simulink model "Wind_turbine_model_L"  (R2020a)
settings: Solver=daessc  StartTime=0.0  StopTime=70  RelTol=1e-3
model workspace (MAT data in the model file):
  Tw : Simulink.Parameter (value not decoded)
  c : Simulink.Parameter (value not decoded)
  r : Simulink.Parameter (value not decoded)
values from neighbouring files (symbols this model uses):
  a1 = 0.5176    [data.mat]
  a2 = 116    [data.mat]
  a3 = 0.4    [data.mat]
  a4 = 5    [data.mat]
  a5 = 21    [data.mat]
  a6 = 0.0068    [data.mat]
  a7 = 0.09    [data.mat]
  a8 = 0.035    [data.mat]
  Ad = 6031.85789489    [data.mat]
  D = 1e-3    (= 0.001)    [Generator_specs.m]
  denp = den_P    [Wind_Turbine_Pitch.m]    (also in data.mat = [91260000000000 145900000000000 1.431e+17 7.554e+15 2.279e+1)
  dent = den_P    [Wind_Turbine_Pitch.m]    (also in data.mat = [91260000000000 145900000000000 1.431e+17 7.554e+15 2.279e+1)
  f = 50    [Generator_specs.m]
  Fs = Vs*sqrt(2/3)/(2*pi*f)    [Generator_specs.m]
  fsw = 4e3    (= 4000)    [Generator_specs.m]
  J = 127/2    (= 63.5)    [Generator_specs.m]
  ki_id = (wn1^2)*Lr*sigma    (= 491.599501999)    [Generator_specs.m]
  ki_n = ((wnn^2)*J)/p    (= 203200)    [Generator_specs.m]
  Kopt = ((0.5*ro*pi*(Radius^5)*cp_max)/(lambda_opt^3))    (= 227539.221001)    [Generator_specs.m]
  kp_id = (2*wn1*sigma*Lr)-Rr    (= 0.5771)    [Generator_specs.m]
  kp_n = (2*wnn*J)/p    (= 5080)    [Generator_specs.m]
  Lm = 2.5e-3    (= 0.0025)    [Generator_specs.m]
  Lr = Lm + Lsi    (= 0.002587)    [Generator_specs.m]
  Ls = Lm + Lsi    (= 0.002587)    [Generator_specs.m]
  Lsi = 0.087e-3    (= 8.7e-05)    [Generator_specs.m]
  N = 100    [Generator_specs.m]
  nump = num_P    [Wind_Turbine_Pitch.m]    (also in data.mat = [16590000 26450000 25540000000 6335000000 3680000000000])
  numt = num_T    [Wind_Turbine_Pitch.m]    (also in data.mat = [-75000000 -527900000000 -306700000000000])
  p = 2    [Generator_specs.m]
  Ps = 2e6    (= 2000000)    [Generator_specs.m]
  Rr = 2.9e-3    (= 0.0029)    [Generator_specs.m]
  Rs = 2.6e-3    (= 0.0026)    [Generator_specs.m]
  s = tf('s')    [Wind_Turbine_Pitch.m]
  sigma = 1 - Lm^2/(Ls*Lr)    (= 0.0661284179513)    [Generator_specs.m]    (also in data.mat = 0.075)
  Tem = 12732    [Generator_specs.m]
  Tgd_max = 14000    [Wind_Turbine_Pitch.m]    (also in data.mat)
  Tie = 1    [data.mat]
  Tiu = 10000    [data.mat]
  Tix = 1    [data.mat]
  Tpe = 1    [data.mat]
  Tpu = 10000    [data.mat]
  Tpx = 10000    [data.mat]
  Ts = 1/fsw/50    (= 5e-06)    [Generator_specs.m]
  Vbus = Vr_stator*sqrt(2)    [Generator_specs.m]
  Vs = 690    [Generator_specs.m]
  WT_Params =     [data.mat]
symbols that are objects in the model workspace (value not decoded): c, r, Tw
undefined symbols (not defined in the file or in its folder): DiscIntNeverNeededParam, sigbuilder_block, X, Y, Z
libraries: sm_lib x21, fl_lib x18, nesl_utility x18, powerlib x8, sdl_lib x3, powerlib_meascontrol x1
(part 2 of 3)

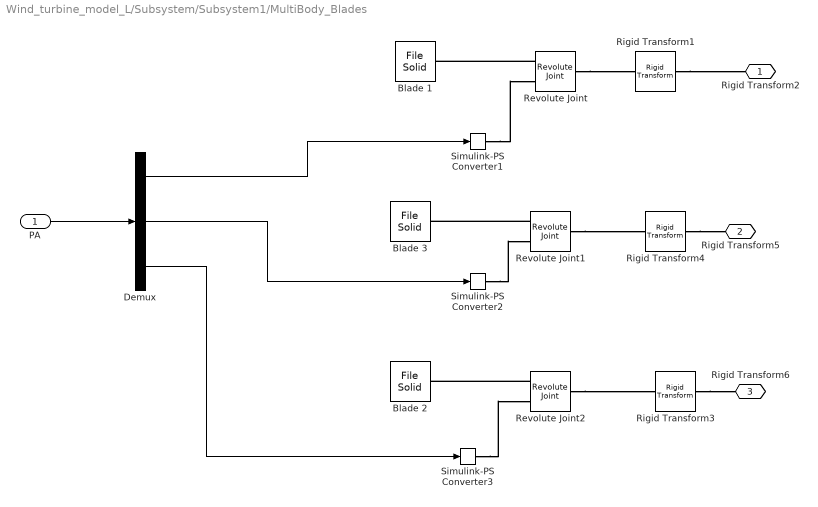
== system Wind_turbine_model_L/Subsystem/Subsystem1/MultiBody_Blades ==
  PA : Inport
  Blade 1 : sm_lib/Body Elements/File Solid  ExtGeomFileName=F:\Altran_Documents\Pilot_Project\Wind_energy\Wind_Turbine_MBSE\Local_WIP\WT blade.STEP  UnitType=FromFile  ExtGeomFileUnits=m  StepReaderType=HEX  ExportConvexHullGeometry=off  InertiaType=PointMass  Mass=5388  MassUnits=kg  CenterOfMass=[0 0 0]  CenterOfMassUnits=m  MomentsOfInertia=[1 1 1]  MomentsOfInertiaUnits=kg*m^2  ProductsOfInertia=[0 0 0]  ProductsOfInertiaUnits=kg*m^2  BasedOnType=DensityFromFile  Density=1000  DensityUnits=kg/m^3  DoExposeReferenceFrame=on  SerializedFrames=<Frames/>  GraphicType=FromGeometry  MarkerShape=Sphere  MarkerSize=10  GraphicVisPropType=SimpleVisualProperties  GraphicDiffuseColor=[0.5 0.5 0.5]  GraphicSpecularColor=[0.5 0.5 0.5 1.0]  GraphicAmbientColor=[0.15 0.15 0.15 1.0]  GraphicEmissiveColor=[0.0 0.0 0.0 1.0]  GraphicShininess=75  GraphicOpacity=1.0
  Blade 2 : sm_lib/Body Elements/File Solid  ExtGeomFileName=F:\Altran_Documents\Pilot_Project\Wind_energy\Wind_Turbine_MBSE\Local_WIP\WT blade.STEP  UnitType=FromFile  ExtGeomFileUnits=m  StepReaderType=HEX  ExportConvexHullGeometry=off  InertiaType=PointMass  Mass=5388  MassUnits=kg  CenterOfMass=[0 0 0]  CenterOfMassUnits=m  MomentsOfInertia=[1 1 1]  MomentsOfInertiaUnits=kg*m^2  ProductsOfInertia=[0 0 0]  ProductsOfInertiaUnits=kg*m^2  BasedOnType=DensityFromFile  Density=1000  DensityUnits=kg/m^3  DoExposeReferenceFrame=on  SerializedFrames=<Frames/>  GraphicType=FromGeometry  MarkerShape=Sphere  MarkerSize=10  GraphicVisPropType=SimpleVisualProperties  GraphicDiffuseColor=[0.5 0.5 0.5]  GraphicSpecularColor=[0.5 0.5 0.5 1.0]  GraphicAmbientColor=[0.15 0.15 0.15 1.0]  GraphicEmissiveColor=[0.0 0.0 0.0 1.0]  GraphicShininess=75  GraphicOpacity=1.0
  Blade 3 : sm_lib/Body Elements/File Solid  ExtGeomFileName=F:\Altran_Documents\Pilot_Project\Wind_energy\Wind_Turbine_MBSE\Local_WIP\WT blade.STEP  UnitType=FromFile  ExtGeomFileUnits=m  StepReaderType=HEX  ExportConvexHullGeometry=off  InertiaType=PointMass  Mass=5388  MassUnits=kg  CenterOfMass=[0 0 0]  CenterOfMassUnits=m  MomentsOfInertia=[1 1 1]  MomentsOfInertiaUnits=kg*m^2  ProductsOfInertia=[0 0 0]  ProductsOfInertiaUnits=kg*m^2  BasedOnType=DensityFromFile  Density=1000  DensityUnits=kg/m^3  DoExposeReferenceFrame=on  SerializedFrames=<Frames/>  GraphicType=FromGeometry  MarkerShape=Sphere  MarkerSize=10  GraphicVisPropType=SimpleVisualProperties  GraphicDiffuseColor=[0.5 0.5 0.5]  GraphicSpecularColor=[0.5 0.5 0.5 1.0]  GraphicAmbientColor=[0.15 0.15 0.15 1.0]  GraphicEmissiveColor=[0.0 0.0 0.0 1.0]  GraphicShininess=75  GraphicOpacity=1.0
  Demux : Demux  Outputs=3
  Revolute Joint : sm_lib/Joints/Revolute Joint  JointMode=Normal  SenseConstraintForce=off  SenseConstraintForceX=off  SenseConstraintForceY=off  SenseConstraintForceZ=off  SenseConstraintTorque=off  SenseConstraintTorqueX=off  SenseConstraintTorqueY=off  SenseConstraintTorqueZ=off  SenseTotalForce=off  SenseTotalForceX=off  SenseTotalForceY=off  SenseTotalForceZ=off  SenseTotalTorque=off  SenseTotalTorqueX=off  SenseTotalTorqueY=off  SenseTotalTorqueZ=off  CompositeWrenchDir=BaseOnFollower  CompositeWrenchFrame=BaseFrame  EquilibriumPosition=0  EquilibriumPositionUnits=deg  SpringStiffness=0  SpringStiffnessUnits=N*m/deg  DampingCoefficient=0  DampingCoefficientUnits=N*m/(deg/s)  TorqueActuationMode=ComputedTorque  MotionActuationMode=InputMotion  SensePosition=off  SenseVelocity=off  SenseAcceleration=off  SenseTorqueForce=off  SenseLowerLimitTorqueForce=off  SenseUpperLimitTorqueForce=off  LowerLimitSpecify=off  LowerLimitBound=-90  LowerLimitBoundUnits=deg  LowerLimitStiffness=1e4  LowerLimitStiffnessUnits=N*m/deg  LowerLimitDamping=10  LowerLimitDampingUnits=N*m/(deg/s)  LowerLimitTransitionRegionWidth=0.1  LowerLimitTransitionRegionWidthUnits=deg  UpperLimitSpecify=off  UpperLimitBound=90  UpperLimitBoundUnits=deg  UpperLimitStiffness=1e4  UpperLimitStiffnessUnits=N*m/deg  UpperLimitDamping=10  UpperLimitDampingUnits=N*m/(deg/s)  UpperLimitTransitionRegionWidth=0.1  UpperLimitTransitionRegionWidthUnits=deg  PositionTargetSpecify=off  PositionTargetPriority=High  PositionTargetValue=30  PositionTargetValueUnits=deg  VelocityTargetSpecify=off  VelocityTargetPriority=High  VelocityTargetValue=0  VelocityTargetValueUnits=deg/s
  Revolute Joint1 : sm_lib/Joints/Revolute Joint  JointMode=Normal  SenseConstraintForce=off  SenseConstraintForceX=off  SenseConstraintForceY=off  SenseConstraintForceZ=off  SenseConstraintTorque=off  SenseConstraintTorqueX=off  SenseConstraintTorqueY=off  SenseConstraintTorqueZ=off  SenseTotalForce=off  SenseTotalForceX=off  SenseTotalForceY=off  SenseTotalForceZ=off  SenseTotalTorque=off  SenseTotalTorqueX=off  SenseTotalTorqueY=off  SenseTotalTorqueZ=off  CompositeWrenchDir=BaseOnFollower  CompositeWrenchFrame=BaseFrame  EquilibriumPosition=0  EquilibriumPositionUnits=deg  SpringStiffness=0  SpringStiffnessUnits=N*m/deg  DampingCoefficient=0  DampingCoefficientUnits=N*m/(deg/s)  TorqueActuationMode=ComputedTorque  MotionActuationMode=InputMotion  SensePosition=off  SenseVelocity=off  SenseAcceleration=off  SenseTorqueForce=off  SenseLowerLimitTorqueForce=off  SenseUpperLimitTorqueForce=off  LowerLimitSpecify=off  LowerLimitBound=-90  LowerLimitBoundUnits=deg  LowerLimitStiffness=1e4  LowerLimitStiffnessUnits=N*m/deg  LowerLimitDamping=10  LowerLimitDampingUnits=N*m/(deg/s)  LowerLimitTransitionRegionWidth=0.1  LowerLimitTransitionRegionWidthUnits=deg  UpperLimitSpecify=off  UpperLimitBound=90  UpperLimitBoundUnits=deg  UpperLimitStiffness=1e4  UpperLimitStiffnessUnits=N*m/deg  UpperLimitDamping=10  UpperLimitDampingUnits=N*m/(deg/s)  UpperLimitTransitionRegionWidth=0.1  UpperLimitTransitionRegionWidthUnits=deg  PositionTargetSpecify=off  PositionTargetPriority=High  PositionTargetValue=30  PositionTargetValueUnits=deg  VelocityTargetSpecify=off  VelocityTargetPriority=High  VelocityTargetValue=0  VelocityTargetValueUnits=deg/s
  Revolute Joint2 : sm_lib/Joints/Revolute Joint  JointMode=Normal  SenseConstraintForce=off  SenseConstraintForceX=off  SenseConstraintForceY=off  SenseConstraintForceZ=off  SenseConstraintTorque=off  SenseConstraintTorqueX=off  SenseConstraintTorqueY=off  SenseConstraintTorqueZ=off  SenseTotalForce=off  SenseTotalForceX=off  SenseTotalForceY=off  SenseTotalForceZ=off  SenseTotalTorque=off  SenseTotalTorqueX=off  SenseTotalTorqueY=off  SenseTotalTorqueZ=off  CompositeWrenchDir=BaseOnFollower  CompositeWrenchFrame=BaseFrame  EquilibriumPosition=0  EquilibriumPositionUnits=deg  SpringStiffness=0  SpringStiffnessUnits=N*m/deg  DampingCoefficient=0  DampingCoefficientUnits=N*m/(deg/s)  TorqueActuationMode=ComputedTorque  MotionActuationMode=InputMotion  SensePosition=off  SenseVelocity=off  SenseAcceleration=off  SenseTorqueForce=off  SenseLowerLimitTorqueForce=off  SenseUpperLimitTorqueForce=off  LowerLimitSpecify=off  LowerLimitBound=-90  LowerLimitBoundUnits=deg  LowerLimitStiffness=1e4  LowerLimitStiffnessUnits=N*m/deg  LowerLimitDamping=10  LowerLimitDampingUnits=N*m/(deg/s)  LowerLimitTransitionRegionWidth=0.1  LowerLimitTransitionRegionWidthUnits=deg  UpperLimitSpecify=off  UpperLimitBound=90  UpperLimitBoundUnits=deg  UpperLimitStiffness=1e4  UpperLimitStiffnessUnits=N*m/deg  UpperLimitDamping=10  UpperLimitDampingUnits=N*m/(deg/s)  UpperLimitTransitionRegionWidth=0.1  UpperLimitTransitionRegionWidthUnits=deg  PositionTargetSpecify=off  PositionTargetPriority=High  PositionTargetValue=30  PositionTargetValueUnits=deg  VelocityTargetSpecify=off  VelocityTargetPriority=High  VelocityTargetValue=0  VelocityTargetValueUnits=deg/s
  Rigid Transform1 : sm_lib/Frames and Transforms/Rigid Transform  TranslationMethod=StandardAxis  TranslationStandardOffset=3.5  TranslationLengthUnit=m  TranslationStandardAxis=+Z  TranslationCartesianOffset=[0 0 0]  TranslationROffset=0  TranslationROffsetUnits=m  TranslationZOffset=0  TranslationZOffsetUnits=m  TranslationThetaOffset=0  TranslationThetaOffsetUnits=deg  RotationMethod=StandardAxis  RotationAngleUnits=deg  RotationStandardAxis=+Z  RotationAngle=180  RotationArbitraryAxis=[0 0 1]  FollAlignAxisA=+X  BaseAlignAxisA=+Y  FollAlignAxisB=+Y  BaseAlignAxisB=+Z  RotationSequenceAxes=FollowerAxes  RotationSequence=XYX  RotationSequenceAngles=[0 0 0]  RotationSequenceAnglesUnits=deg  RotationMatrix=[1 0 0; 0 1 0; 0 0 1]
  Rigid Transform3 : sm_lib/Frames and Transforms/Rigid Transform  TranslationMethod=StandardAxis  TranslationStandardOffset=3.5  TranslationLengthUnit=m  TranslationStandardAxis=-Z  TranslationCartesianOffset=[0 0 0]  TranslationROffset=0  TranslationROffsetUnits=m  TranslationZOffset=0  TranslationZOffsetUnits=m  TranslationThetaOffset=0  TranslationThetaOffsetUnits=deg  RotationMethod=StandardAxis  RotationAngleUnits=deg  RotationStandardAxis=+Y  RotationAngle=30  RotationArbitraryAxis=[0 0 1]  FollAlignAxisA=+X  BaseAlignAxisA=+Y  FollAlignAxisB=+Y  BaseAlignAxisB=+Z  RotationSequenceAxes=FollowerAxes  RotationSequence=XYX  RotationSequenceAngles=[0 0 0]  RotationSequenceAnglesUnits=deg  RotationMatrix=[1 0 0; 0 1 0; 0 0 1]
  Rigid Transform4 : sm_lib/Frames and Transforms/Rigid Transform  TranslationMethod=StandardAxis  TranslationStandardOffset=3.5  TranslationLengthUnit=m  TranslationStandardAxis=-Z  TranslationCartesianOffset=[0 0 0]  TranslationROffset=0  TranslationROffsetUnits=m  TranslationZOffset=0  TranslationZOffsetUnits=m  TranslationThetaOffset=0  TranslationThetaOffsetUnits=deg  RotationMethod=StandardAxis  RotationAngleUnits=deg  RotationStandardAxis=-Y  RotationAngle=30  RotationArbitraryAxis=[0 0 1]  FollAlignAxisA=+X  BaseAlignAxisA=+Y  FollAlignAxisB=+Y  BaseAlignAxisB=+Z  RotationSequenceAxes=FollowerAxes  RotationSequence=XYX  RotationSequenceAngles=[0 0 0]  RotationSequenceAnglesUnits=deg  RotationMatrix=[1 0 0; 0 1 0; 0 0 1]
  Simulink-PS Converter1 : nesl_utility/Simulink-PS Converter  PhysicalDomain=network_engine_domain  SubClassName=ps_input  LeftPortType=input  RightPortType=output  PseudoPeriodic=off  Frequencies=[]  NoiseDistribution=none  NoiseParameters=[]  Unit=1  AffineConversion=off  FilteringAndDerivatives=filter  SimscapeFilterOrder=2  InputFilterTimeConstant=0.001  UdotUserProvided=0
      settings: SourceProductBaseCode=MT,SS
  Simulink-PS Converter2 : nesl_utility/Simulink-PS Converter  PhysicalDomain=network_engine_domain  SubClassName=ps_input  LeftPortType=input  RightPortType=output  PseudoPeriodic=off  Frequencies=[]  NoiseDistribution=none  NoiseParameters=[]  Unit=1  AffineConversion=off  FilteringAndDerivatives=filter  SimscapeFilterOrder=2  InputFilterTimeConstant=0.001  UdotUserProvided=0
      settings: SourceProductBaseCode=MT,SS
  Simulink-PS Converter3 : nesl_utility/Simulink-PS Converter  PhysicalDomain=network_engine_domain  SubClassName=ps_input  LeftPortType=input  RightPortType=output  PseudoPeriodic=off  Frequencies=[]  NoiseDistribution=none  NoiseParameters=[]  Unit=1  AffineConversion=off  FilteringAndDerivatives=filter  SimscapeFilterOrder=2  InputFilterTimeConstant=0.001  UdotUserProvided=0
      settings: SourceProductBaseCode=MT,SS
  Rigid Transform2 : PMIOPort  Side=Right
  Rigid Transform5 : PMIOPort  Port=2  Side=Right
  Rigid Transform6 : PMIOPort  Port=3  Side=Right
  wires:
  Demux/1 -> Simulink-PS Converter1/1
  Demux/3 -> Simulink-PS Converter3/1
  Demux/2 -> Simulink-PS Converter2/1
  PA/1 -> Demux/1
  connections:
  Rigid Transform4/RConn1 -- Rigid Transform5/RConn1
  Revolute Joint2/LConn1 -- Blade 2/RConn1
  Simulink-PS Converter3/RConn1 -- Revolute Joint2/LConn2
  Revolute Joint1/RConn1 -- Rigid Transform4/LConn1
  Revolute Joint2/RConn1 -- Rigid Transform3/LConn1
  Revolute Joint/RConn1 -- Rigid Transform1/RConn1
  Simulink-PS Converter2/RConn1 -- Revolute Joint1/LConn2
  Revolute Joint1/LConn1 -- Blade 3/RConn1
  Rigid Transform1/LConn1 -- Rigid Transform2/RConn1
  Revolute Joint/LConn1 -- Blade 1/RConn1
  Simulink-PS Converter1/RConn1 -- Revolute Joint/LConn2
  Rigid Transform3/RConn1 -- Rigid Transform6/RConn1

== system Wind_turbine_model_L/Subsystem/Subsystem1/Nacelle ==
  Ideal Actuator : Subsystem  AncestorBlock=Yaw_Actuation_Lib/Ideal Actuator
      mask Display: image('Yaw_Ideal_Actuation_IMAGE.jpg');
  Mux : Mux  Inputs=2
  Nacelle : sm_lib/Body Elements/File Solid  ExtGeomFileName=F:\Altran_Documents\Pilot_Project\Wind_energy\Wind_Turbine_MBSE\Local_WIP\WT nacelle.STEP  UnitType=FromFile  ExtGeomFileUnits=m  StepReaderType=HEX  ExportConvexHullGeometry=off  InertiaType=PointMass  Mass=56310  MassUnits=kg  CenterOfMass=[0 0 0]  CenterOfMassUnits=m  MomentsOfInertia=[1 1 1]  MomentsOfInertiaUnits=kg*m^2  ProductsOfInertia=[0 0 0]  ProductsOfInertiaUnits=kg*m^2  BasedOnType=DensityFromFile  Density=1000  DensityUnits=kg/m^3  DoExposeReferenceFrame=on  SerializedFrames=<Frames><Frame><Id>Frame1</Id><Value><Name>T</Name><Origin><Source>GeometricFeature</Source><FeatureName>circular curve 2</FeatureName></Origin><PrimaryAxis><DefinedDirection>+Z</DefinedDirection><Source>ReferenceFrame</Source><SourceDirection>+Z</SourceDirection><FeatureName></FeatureName></PrimaryAxis><SecondaryAxis><DefinedDirection>+X</DefinedDirection><Source>ReferenceFrame</Source><SourceDirection>+X</SourceDirection><FeatureName></FeatureName></SecondaryAxis></Value></Frame></Frames>  GraphicType=FromGeometry  MarkerShape=Sphere  MarkerSize=10  GraphicVisPropType=SimpleVisualProperties  GraphicDiffuseColor=[0.5 0.5 0.5]  GraphicSpecularColor=[0.5 0.5 0.5 1.0]  GraphicAmbientColor=[0.15 0.15 0.15 1.0]  GraphicEmissiveColor=[0.0 0.0 0.0 1.0]  GraphicShininess=75  GraphicOpacity=1.0
  PS-Simulink Converter : nesl_utility/PS-Simulink Converter  PhysicalDomain=network_engine_domain  SubClassName=ps_output  LeftPortType=input  RightPortType=output  PseudoPeriodic=off  Frequencies=[]  Unit=deg  AffineConversion=off
  PS-Simulink Converter1 : nesl_utility/PS-Simulink Converter  PhysicalDomain=network_engine_domain  SubClassName=ps_output  LeftPortType=input  RightPortType=output  PseudoPeriodic=off  Frequencies=[]  Unit=deg/s  AffineConversion=off
  Revolute Joint4 : sm_lib/Joints/Revolute Joint  JointMode=Normal  SenseConstraintForce=off  SenseConstraintForceX=off  SenseConstraintForceY=off  SenseConstraintForceZ=off  SenseConstraintTorque=off  SenseConstraintTorqueX=off  SenseConstraintTorqueY=off  SenseConstraintTorqueZ=off  SenseTotalForce=off  SenseTotalForceX=off  SenseTotalForceY=off  SenseTotalForceZ=off  SenseTotalTorque=off  SenseTotalTorqueX=off  SenseTotalTorqueY=off  SenseTotalTorqueZ=off  CompositeWrenchDir=FollowerOnBase  CompositeWrenchFrame=BaseFrame  EquilibriumPosition=0  EquilibriumPositionUnits=deg  SpringStiffness=0  SpringStiffnessUnits=N*m/deg  DampingCoefficient=0  DampingCoefficientUnits=N*m/(deg/s)  TorqueActuationMode=InputTorque  MotionActuationMode=ComputedMotion  SensePosition=on  SenseVelocity=on  SenseAcceleration=off  SenseTorqueForce=off  SenseLowerLimitTorqueForce=off  SenseUpperLimitTorqueForce=off  LowerLimitSpecify=off  LowerLimitBound=0  LowerLimitBoundUnits=deg  LowerLimitStiffness=1e4  LowerLimitStiffnessUnits=N*m/deg  LowerLimitDamping=10  LowerLimitDampingUnits=N*m/(deg/s)  LowerLimitTransitionRegionWidth=0.1  LowerLimitTransitionRegionWidthUnits=deg  UpperLimitSpecify=off  UpperLimitBound=120  UpperLimitBoundUnits=deg  UpperLimitStiffness=1e4  UpperLimitStiffnessUnits=N*m/deg  UpperLimitDamping=10  UpperLimitDampingUnits=N*m/(deg/s)  UpperLimitTransitionRegionWidth=0.1  UpperLimitTransitionRegionWidthUnits=deg  PositionTargetSpecify=off  PositionTargetPriority=High  PositionTargetValue=30  PositionTargetValueUnits=deg  VelocityTargetSpecify=off  VelocityTargetPriority=High  VelocityTargetValue=0  VelocityTargetValueUnits=deg/s
  Rigid Transform : sm_lib/Frames and Transforms/Rigid Transform  TranslationMethod=StandardAxis  TranslationStandardOffset=4.5  TranslationLengthUnit=m  TranslationStandardAxis=+Z  TranslationCartesianOffset=[0 0 0]  TranslationROffset=0  TranslationROffsetUnits=m  TranslationZOffset=0  TranslationZOffsetUnits=m  TranslationThetaOffset=0  TranslationThetaOffsetUnits=deg  RotationMethod=None  RotationAngleUnits=deg  RotationStandardAxis=+Z  RotationAngle=0.0  RotationArbitraryAxis=[0 0 1]  FollAlignAxisA=+X  BaseAlignAxisA=+Y  FollAlignAxisB=+Y  BaseAlignAxisB=+Z  RotationSequenceAxes=FollowerAxes  RotationSequence=XYX  RotationSequenceAngles=[0 0 0]  RotationSequenceAnglesUnits=deg  RotationMatrix=[1 0 0; 0 1 0; 0 0 1]
  Rigid Transform6 : sm_lib/Frames and Transforms/Rigid Transform  TranslationMethod=None  TranslationStandardOffset=4.5  TranslationLengthUnit=m  TranslationStandardAxis=-Z  TranslationCartesianOffset=[0 0 0]  TranslationROffset=0  TranslationROffsetUnits=m  TranslationZOffset=0  TranslationZOffsetUnits=m  TranslationThetaOffset=0  TranslationThetaOffsetUnits=deg  RotationMethod=AlignedAxes  RotationAngleUnits=deg  RotationStandardAxis=+Z  RotationAngle=0.0  RotationArbitraryAxis=[0 0 1]  FollAlignAxisA=+Z  BaseAlignAxisA=+Y  FollAlignAxisB=+X  BaseAlignAxisB=+X  RotationSequenceAxes=FollowerAxes  RotationSequence=XYX  RotationSequenceAngles=[0 0 0]  RotationSequenceAnglesUnits=deg  RotationMatrix=[1 0 0; 0 1 0; 0 0 1]
  Simulink-PS Converter : nesl_utility/Simulink-PS Converter  PhysicalDomain=network_engine_domain  SubClassName=ps_input  LeftPortType=input  RightPortType=output  PseudoPeriodic=off  Frequencies=[]  NoiseDistribution=none  NoiseParameters=[]  Unit=1  AffineConversion=off  FilteringAndDerivatives=provide  SimscapeFilterOrder=1  InputFilterTimeConstant=0.001  UdotUserProvided=0
  Two-Way Connection : TwoWayConnection
  Rigid Transform1 : PMIOPort  Side=Left
  Revolute Joint1 : PMIOPort  Port=2  Side=Left
  YC : PMIOPort  Port=3  Side=Left
  wires:
  PS-Simulink Converter1/1 -> Mux/2
  PS-Simulink Converter/1 -> Mux/1
  Mux/1 -> Two-Way Connection/1
  Two-Way Connection/1 -> Simulink-PS Converter/1
  connections:
  Rigid Transform6/RConn1 -- Revolute Joint4/RConn1
  Rigid Transform6/LConn1 -- Nacelle/LConn1
  Revolute Joint1/RConn1 -- Revolute Joint4/LConn1
  Nacelle/RConn1 -- Rigid Transform/LConn1
  PS-Simulink Converter/LConn1 -- Revolute Joint4/RConn2
  Rigid Transform/RConn1 -- Rigid Transform1/RConn1
  YC/RConn1 -- Ideal Actuator/RConn1
  Simulink-PS Converter/RConn1 -- Revolute Joint4/LConn2
  PS-Simulink Converter1/LConn1 -- Revolute Joint4/RConn3
  Two-Way Connection/RConn1 -- Ideal Actuator/LConn1

== system Wind_turbine_model_L/Subsystem/Subsystem1/Subsystem ==
  Ang_Vel_PS-Simulink Converter1 : nesl_utility/PS-Simulink Converter  PhysicalDomain=network_engine_domain  SubClassName=ps_output  LeftPortType=input  RightPortType=output  PseudoPeriodic=off  Frequencies=[]  Unit=inherit  AffineConversion=off
      settings: SourceProductBaseCode=MT,SS
  Ang_Vel_PS-Simulink Converter3 : nesl_utility/PS-Simulink Converter  PhysicalDomain=network_engine_domain  SubClassName=ps_output  LeftPortType=input  RightPortType=output  PseudoPeriodic=off  Frequencies=[]  Unit=inherit  AffineConversion=off
      settings: SourceProductBaseCode=MT,SS
  Hub : sm_lib/Body Elements/File Solid  ExtGeomFileName=F:\Altran_Documents\Pilot_Project\Wind_energy\Wind_Turbine_MBSE\Local_WIP\WT hub.STEP  UnitType=FromFile  ExtGeomFileUnits=m  StepReaderType=HEX  ExportConvexHullGeometry=off  InertiaType=PointMass  Mass=18770  MassUnits=kg  CenterOfMass=[0 0 0]  CenterOfMassUnits=m  MomentsOfInertia=[1 1 1]  MomentsOfInertiaUnits=kg*m^2  ProductsOfInertia=[0 0 0]  ProductsOfInertiaUnits=kg*m^2  BasedOnType=DensityFromFile  Density=1000  DensityUnits=kg/m^3  DoExposeReferenceFrame=on  SerializedFrames=<Frames><Frame><Id>Frame1</Id><Value><Name>B1</Name><Origin><Source>GeometricFeature</Source><FeatureName>circular curve 23</FeatureName></Origin><PrimaryAxis><DefinedDirection>+Z</DefinedDirection><Source>ReferenceFrame</Source><SourceDirection>+Y</SourceDirection><FeatureName></FeatureName></PrimaryAxis><SecondaryAxis><DefinedDirection>+X</DefinedDirection><Source>ReferenceFrame</Source><SourceDirection>+X</SourceDirection><FeatureName></FeatureName></SecondaryAxis></Value></Frame><Frame><Id>Frame3</Id><Value><Name>B3</Name><Origin><Source>GeometricFeature</Source><FeatureName>circular curve 21</FeatureName></Origin><PrimaryAxis><DefinedDirection>+Z</DefinedDirection><Source>ReferenceFrame</Source><SourceDirection>-X</SourceDirection><FeatureName></FeatureName></PrimaryAxis><SecondaryAxis><DefinedDirection>+X</DefinedDirection><Source>ReferenceFrame</Source><SourceDirection>-Y</SourceDirection><FeatureName></FeatureName></SecondaryAxis></Value></Frame><Frame><Id>Frame4</Id><Value><Name>B2</Name><Origin><Source>GeometricFeature</Source><FeatureName>circular curve 25</FeatureName></Origin><PrimaryAxis><DefinedDirection>+Z</DefinedDirection><Source>ReferenceFrame</Source><SourceDirection>+X</SourceDirection><FeatureName></FeatureName></PrimaryAxis><SecondaryAxis><DefinedDirection>+X</DefinedDirection><Source>ReferenceFrame</Source><SourceDirection>+Y</SourceDirection><FeatureName></FeatureName></SecondaryAxis></Value></Frame></Frames>  GraphicType=FromGeometry  MarkerShape=Sphere  MarkerSize=10  GraphicVisPropType=SimpleVisualProperties  GraphicDiffuseColor=[0.5 0.5 0.5]  GraphicSpecularColor=[0.5 0.5 0.5 1.0]  GraphicAmbientColor=[0.15 0.15 0.15 1.0]  GraphicEmissiveColor=[0.0 0.0 0.0 1.0]  GraphicShininess=75  GraphicOpacity=1.0
  Revolute Joint3 : sm_lib/Joints/Revolute Joint  JointMode=Normal  SenseConstraintForce=off  SenseConstraintForceX=off  SenseConstraintForceY=off  SenseConstraintForceZ=off  SenseConstraintTorque=off  SenseConstraintTorqueX=off  SenseConstraintTorqueY=off  SenseConstraintTorqueZ=off  SenseTotalForce=off  SenseTotalForceX=off  SenseTotalForceY=off  SenseTotalForceZ=off  SenseTotalTorque=off  SenseTotalTorqueX=off  SenseTotalTorqueY=off  SenseTotalTorqueZ=off  CompositeWrenchDir=FollowerOnBase  CompositeWrenchFrame=BaseFrame  EquilibriumPosition=0  EquilibriumPositionUnits=deg  SpringStiffness=0  SpringStiffnessUnits=N*m/deg  DampingCoefficient=0  DampingCoefficientUnits=N*m/(deg/s)  TorqueActuationMode=InputTorque  MotionActuationMode=ComputedMotion  SensePosition=off  SenseVelocity=on  SenseAcceleration=off  SenseTorqueForce=on  SenseLowerLimitTorqueForce=off  SenseUpperLimitTorqueForce=off  LowerLimitSpecify=off  LowerLimitBound=-90  LowerLimitBoundUnits=deg  LowerLimitStiffness=1e4  LowerLimitStiffnessUnits=N*m/deg  LowerLimitDamping=10  LowerLimitDampingUnits=N*m/(deg/s)  LowerLimitTransitionRegionWidth=0.1  LowerLimitTransitionRegionWidthUnits=deg  UpperLimitSpecify=off  UpperLimitBound=90  UpperLimitBoundUnits=deg  UpperLimitStiffness=1e4  UpperLimitStiffnessUnits=N*m/deg  UpperLimitDamping=10  UpperLimitDampingUnits=N*m/(deg/s)  UpperLimitTransitionRegionWidth=0.1  UpperLimitTransitionRegionWidthUnits=deg  PositionTargetSpecify=off  PositionTargetPriority=High  PositionTargetValue=0  PositionTargetValueUnits=deg  VelocityTargetSpecify=off  VelocityTargetPriority=High  VelocityTargetValue=0  VelocityTargetValueUnits=deg/s
  Rotor_Ang_Vel : Scope
  Rotor_Torque : Scope
  Blade2 : PMIOPort  Side=Left
  Blade1 : PMIOPort  Port=2  Side=Left
  Blade3 : PMIOPort  Port=3  Side=Left
  Spinning_Torque : PMIOPort  Port=4  Side=Left
  Nacelle : PMIOPort  Port=5  Side=Right
  wires:
  Ang_Vel_PS-Simulink Converter3/1 -> Rotor_Torque/1
  Ang_Vel_PS-Simulink Converter1/1 -> Rotor_Ang_Vel/1
  connections:
  Nacelle/RConn1 -- Revolute Joint3/LConn1
  Ang_Vel_PS-Simulink Converter3/LConn1 -- Revolute Joint3/RConn3
  Revolute Joint3/RConn2 -- Ang_Vel_PS-Simulink Converter1/LConn1
  Revolute Joint3/RConn1 -- Hub/RConn1
  Blade3/RConn1 -- Hub/RConn2
  Revolute Joint3/LConn2 -- Spinning_Torque/RConn1
  Blade1/RConn1 -- Hub/LConn2
  Blade2/RConn1 -- Hub/LConn1

== system Wind_turbine_model_L/Subsystem/Subsystem1/Tower ==
  Mechanism Configuration : sm_lib/Utilities/Mechanism Configuration  UniformGravity=Constant  GravityVector=[0 -9.80665 0]  GravityUnits=m/s^2  LinearizationDelta=0.001
  Reaction_PS-Simulink Converter : nesl_utility/PS-Simulink Converter  PhysicalDomain=network_engine_domain  SubClassName=ps_output  LeftPortType=input  RightPortType=output  PseudoPeriodic=off  Frequencies=[]  Unit=inherit  AffineConversion=off
      settings: SourceProductBaseCode=MT,SS
  Reaction_PS-Simulink Converter1 : nesl_utility/PS-Simulink Converter  PhysicalDomain=network_engine_domain  SubClassName=ps_output  LeftPortType=input  RightPortType=output  PseudoPeriodic=off  Frequencies=[]  Unit=inherit  AffineConversion=off
      settings: SourceProductBaseCode=MT,SS
  Rigid Transform2 : sm_lib/Frames and Transforms/Rigid Transform  TranslationMethod=None  TranslationStandardOffset=4.5  TranslationLengthUnit=m  TranslationStandardAxis=-Z  TranslationCartesianOffset=[0 0 0]  TranslationROffset=0  TranslationROffsetUnits=m  TranslationZOffset=0  TranslationZOffsetUnits=m  TranslationThetaOffset=0  TranslationThetaOffsetUnits=deg  RotationMethod=AlignedAxes  RotationAngleUnits=deg  RotationStandardAxis=+Z  RotationAngle=0.0  RotationArbitraryAxis=[0 0 1]  FollAlignAxisA=+Z  BaseAlignAxisA=+Y  FollAlignAxisB=+X  BaseAlignAxisB=+X  RotationSequenceAxes=FollowerAxes  RotationSequence=XYX  RotationSequenceAngles=[0 0 0]  RotationSequenceAnglesUnits=deg  RotationMatrix=[1 0 0; 0 1 0; 0 0 1]
  Rigid Transform5 : sm_lib/Frames and Transforms/Rigid Transform  TranslationMethod=None  TranslationStandardOffset=4.5  TranslationLengthUnit=m  TranslationStandardAxis=-Z  TranslationCartesianOffset=[0 0 0]  TranslationROffset=0  TranslationROffsetUnits=m  TranslationZOffset=0  TranslationZOffsetUnits=m  TranslationThetaOffset=0  TranslationThetaOffsetUnits=deg  RotationMethod=None  RotationAngleUnits=deg  RotationStandardAxis=+Z  RotationAngle=0.0  RotationArbitraryAxis=[0 0 1]  FollAlignAxisA=+X  BaseAlignAxisA=+Y  FollAlignAxisB=+Y  BaseAlignAxisB=+Z  RotationSequenceAxes=FollowerAxes  RotationSequence=XYX  RotationSequenceAngles=[0 0 0]  RotationSequenceAnglesUnits=deg  RotationMatrix=[1 0 0; 0 1 0; 0 0 1]
  Solver Configuration : nesl_utility/Solver Configuration  PhysicalDomain=network_engine_domain  SubClassName=solver  LeftPortType=input  RightPortType=generic  Tones=[]  Harmonics=[]  SimulateNoise=off  Profile=off  UseLocalSampling=off  EnableSwitchedLinearOptims=on  FrequencyDomain=off  UseCCode=off  RelTol=0.001  AbsTol=1e-06  MinStep=1e-09  ToWorkspace=off  RevertToSquareIcSolve=off  NumHomotopyIterations=100  PhasorMode=off  PhasorModeNumHarmonics=1  DoDC=off  ResidualTolerance=1e-09  UseLocalSolver=off  LocalSolverChoice=NE_BACKWARD_EULER_ADVANCER  LocalSolverSampleTime=0.001  DoFixedCost=off  MaxNonlinIter=3  MaxModeIter=2  LinearAlgebra=Sparse  EquationFormulation=NE_TIME_EF  DelaysMemoryBudget=1024  AutomaticFiltering=on  FilteringTimeConstant=0.001  PartitionStorageMethod=AS_NEEDED  PartitionMemoryBudget=1024  PartitionMethod=FAST
      settings: SourceProductBaseCode=MT,SS
  Tower : sm_lib/Body Elements/File Solid  ExtGeomFileName=F:\Altran_Documents\Pilot_Project\Wind_energy\Wind_Turbine_MBSE\Local_WIP\WT tower.STEP  UnitType=FromFile  ExtGeomFileUnits=m  StepReaderType=HEX  ExportConvexHullGeometry=off  InertiaType=PointMass  Mass=115614.8  MassUnits=kg  CenterOfMass=[0 0 0]  CenterOfMassUnits=m  MomentsOfInertia=[1 1 1]  MomentsOfInertiaUnits=kg*m^2  ProductsOfInertia=[0 0 0]  ProductsOfInertiaUnits=kg*m^2  BasedOnType=DensityFromFile  Density=1000  DensityUnits=kg/m^3  DoExposeReferenceFrame=on  SerializedFrames=<Frames><Frame><Id>Frame1</Id><Value><Name>F1</Name><Origin><Source>GeometricFeature</Source><FeatureName>circular curve 3</FeatureName></Origin><PrimaryAxis><DefinedDirection>+Y</DefinedDirection><Source>ReferenceFrame</Source><SourceDirection>+Y</SourceDirection><FeatureName></FeatureName></PrimaryAxis><SecondaryAxis><DefinedDirection>+X</DefinedDirection><Source>ReferenceFrame</Source><SourceDirection>+X</SourceDirection><FeatureName></FeatureName></SecondaryAxis></Value></Frame></Frames>  GraphicType=FromGeometry  MarkerShape=Sphere  MarkerSize=10  GraphicVisPropType=SimpleVisualProperties  GraphicDiffuseColor=[0.5 0.5 0.5]  GraphicSpecularColor=[0.5 0.5 0.5 1.0]  GraphicAmbientColor=[0.15 0.15 0.15 1.0]  GraphicEmissiveColor=[0.0 0.0 0.0 1.0]  GraphicShininess=75  GraphicOpacity=1.0
  Tower_Base_Moment : Scope
  Tower_Base_Reaction : Scope
  Weld Joint : sm_lib/Joints/Weld Joint  JointMode=Normal  SenseConstraintForce=off  SenseConstraintForceX=off  SenseConstraintForceY=off  SenseConstraintForceZ=off  SenseConstraintTorque=off  SenseConstraintTorqueX=off  SenseConstraintTorqueY=off  SenseConstraintTorqueZ=off  SenseTotalForce=on  SenseTotalForceX=off  SenseTotalForceY=off  SenseTotalForceZ=off  SenseTotalTorque=on  SenseTotalTorqueX=off  SenseTotalTorqueY=off  SenseTotalTorqueZ=off  CompositeWrenchDir=FollowerOnBase  CompositeWrenchFrame=BaseFrame
  World Frame : sm_lib/Frames and Transforms/World Frame
  Rigid Transform1 : PMIOPort  Side=Right
  wires:
  Reaction_PS-Simulink Converter/1 -> Tower_Base_Reaction/1
  Reaction_PS-Simulink Converter1/1 -> Tower_Base_Moment/1
  connections:
  Mechanism Configuration/RConn1 -- Solver Configuration/RConn1 -- Weld Joint/LConn1 -- World Frame/RConn1
  Weld Joint/RConn2 -- Reaction_PS-Simulink Converter/LConn1
  Weld Joint/RConn3 -- Reaction_PS-Simulink Converter1/LConn1
  Rigid Transform5/RConn1 -- Tower/LConn1
  Weld Joint/RConn1 -- Rigid Transform5/LConn1
  Rigid Transform2/LConn1 -- Tower/RConn1
  Rigid Transform2/RConn1 -- Rigid Transform1/RConn1

== system Wind_turbine_model_L/Subsystem/Yaw Controller/Yaw Controller ==
  Yaw Command : Inport
  Yaw Rate : Inport  Port=2
  Yaw : Inport  Port=3
  Derivative Control : Gain  Gain=WT_Params.Yaw_Controller.D_Gain*0
  Limit Nacelle Yaw Rate Cmd : Saturate  UpperLimit=WT_Params.Yaw_Actuator.max_yaw_rate  LowerLimit=-WT_Params.Yaw_Actuator.max_yaw_rate
  Limit Servomotor Torque Cmd : Saturate  UpperLimit=max(WT_Params.Yaw_Actuator.Motor.max_torque_vector)  LowerLimit=-max(WT_Params.Yaw_Actuator.Motor.max_torque_vector)
  PI Controller Nacelle Yaw : Subsystem
  PI Controller Nacelle Yaw Rate : Subsystem
  Sum : Sum  Inputs=|+-
  Sum1 : Sum  Inputs=|+-
  Sum3 : Sum  Inputs=|++
  Torque Command : Outport  VectorParamsAs1DForOutWhenUnconnected=off
  tag scope: Yaw_Command=global
  wires:
  Limit Servomotor Torque Cmd/1 -> Torque Command/1  "Torque Command"
  Yaw Rate/1 -> Derivative Control/1, Sum1/2
  Yaw/1 -> Sum3/1
  Sum/1 -> PI Controller Nacelle Yaw/1(e)
  Yaw Command/1 -> Sum/1, [Yaw_Command]
  Sum3/1 -> Sum/2
  Derivative Control/1 -> Sum3/2
  Limit Nacelle Yaw Rate Cmd/1 -> Sum1/1
  Sum1/1 -> PI Controller Nacelle Yaw Rate/1(e)
  PI Controller Nacelle Yaw/1(u) -> Limit Nacelle Yaw Rate Cmd/1
  PI Controller Nacelle Yaw Rate/1(u) -> Limit Servomotor Torque Cmd/1

== system Wind_turbine_model_L/Generator/Controller/Subsystem/D//Q-->alfa//beta ==
  abc : Inport
  Fcn : Fcn  Expr=2/3*(u[1]-u[2]/2-u[3]/2)
  Fcn1 : Fcn  Expr=2/3*(u[2]*(sqrt(3)/2)-u[3]*(sqrt(3)/2))
  Mux : Mux  Inputs=2
  alfa/beta : Outport
  wires:
  Mux/1 -> alfa/beta/1
  Fcn1/1 -> Mux/2
  Fcn/1 -> Mux/1
  abc/1 -> Fcn/1, Fcn1/1

== system Wind_turbine_model_L/Rotor&Pitch_Control/Wr Plant/Wind Turbine/cp(lambda,beta) ==
  lambda : Inport
  beta : Inport  Port=2
  Fcn : Fcn  Expr=1/(1/(u[1]+a7*u[2])-a8/(u[2]^3+1))
  Fcn1 : Fcn  Expr=a1*(a2/u[2]-a3*u[3]-a4)*exp(-a5/u[2])+a6*u[1]
  Mux : Mux  Inputs=2
  Mux1 : Mux  Inputs=3
  cp : Outport
  wires:
  Mux/1 -> Fcn/1
  beta/1 -> Mux/2, Mux1/3
  Mux1/1 -> Fcn1/1
  lambda/1 -> Mux/1, Mux1/1
  Fcn1/1 -> cp/1
  Fcn/1 -> Mux1/2  "lambda_i"

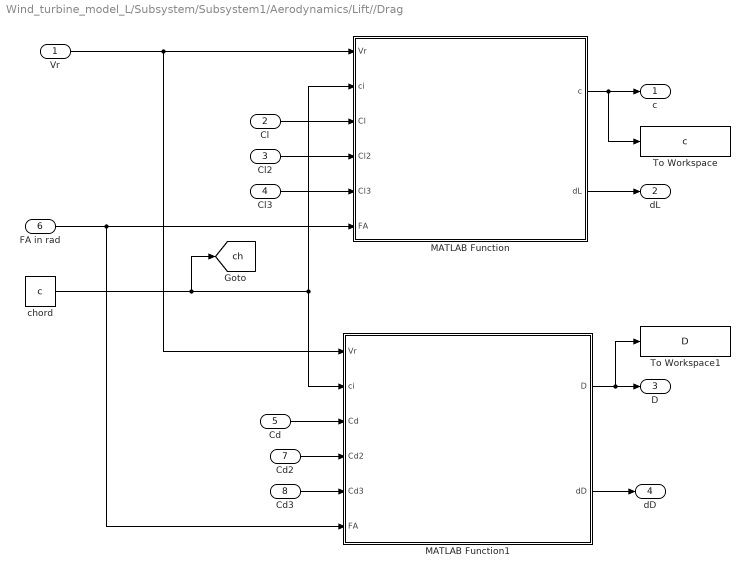
== system Wind_turbine_model_L/Subsystem/Subsystem1/Aerodynamics/Lift//Drag ==
  Vr : Inport
  Cl : Inport  Port=2
  Cl2 : Inport  Port=3
  Cl3 : Inport  Port=4
  Cd : Inport  Port=5
  FA in rad : Inport  Port=6
  Cd2 : Inport  Port=7
  Cd3 : Inport  Port=8
  MATLAB Function : MATLAB Function  TreatAsAtomicUnit=on
  MATLAB Function1 : MATLAB Function  TreatAsAtomicUnit=on
  To Workspace : ToWorkspace  VariableName=c  SampleTime=-1
      settings: Save2DSignal=2-D array (concatenate along first dimension)
  To Workspace1 : ToWorkspace  VariableName=D  SampleTime=-1
      settings: Save2DSignal=2-D array (concatenate along first dimension)
  chord : Constant  Value=c
  c : Outport
  dL : Outport  Port=2
  D : Outport  Port=3
  dD : Outport  Port=4
  tag scope: ch=global
  wires:
  Cl2/1 -> MATLAB Function/4(Cl2)
  Cl/1 -> MATLAB Function/3(Cl)
  FA in rad/1 -> MATLAB Function1/6(FA), MATLAB Function/6(FA)
  Cd3/1 -> MATLAB Function1/5(Cd3)
  chord/1 -> MATLAB Function1/2(ci), MATLAB Function/2(ci), [ch]
  MATLAB Function/2(dL) -> dL/1
  Vr/1 -> MATLAB Function1/1(Vr), MATLAB Function/1(Vr)
  Cd2/1 -> MATLAB Function1/4(Cd2)
  Cl3/1 -> MATLAB Function/5(Cl3)
  Cd/1 -> MATLAB Function1/3(Cd)
  MATLAB Function1/2(dD) -> dD/1
  MATLAB Function1/1(D) -> To Workspace1/1, D/1
  MATLAB Function/1(c) -> To Workspace/1, c/1

== system Wind_turbine_model_L/Subsystem/Subsystem1/Aerodynamics/LookUp_Table ==
  AOA : Inport
  FFAW3_241(9to17) : Subsystem
  FFAW3_301(3to8) : Subsystem
  NACA _63-415(18to25) : Subsystem
  To Workspace : ToWorkspace  VariableName=Cl  SampleTime=-1
      settings: Save2DSignal=2-D array (concatenate along first dimension)
  To Workspace1 : ToWorkspace  VariableName=Cl2  SampleTime=-1
      settings: Save2DSignal=2-D array (concatenate along first dimension)
  Cl : Outport
  Cl2 : Outport  Port=2
  Cl3 : Outport  Port=3
  Cd : Outport  Port=4
  Cd2 : Outport  Port=5
  Cd3 : Outport  Port=6
  wires:
  FFAW3_301(3to8)/2(Output1) -> Cd/1
  AOA/1 -> NACA _63-415(18to25)/1(AOA), FFAW3_241(9to17)/1(AOA), FFAW3_301(3to8)/1(In1)
  FFAW3_301(3to8)/1(Output) -> To Workspace/1, Cl/1
  FFAW3_241(9to17)/1(Output) -> To Workspace1/1, Cl2/1
  FFAW3_241(9to17)/2(Output1) -> Cd2/1
  NACA _63-415(18to25)/1(Output) -> Cl3/1
  NACA _63-415(18to25)/2(Output1) -> Cd3/1

== system Wind_turbine_model_L/Subsystem/Subsystem1/Aerodynamics/Torque ==
  dL : Inport
  dD : Inport  Port=2
  r : Inport  Port=3
  Product1 : Product
  Sum1 : Sum  Inputs=|+-
  To Workspace1 : ToWorkspace  VariableName=TotalTorque  SampleTime=-1
      settings: Save2DSignal=2-D array (concatenate along first dimension)
  To Workspace7 : ToWorkspace  VariableName=dQ  SampleTime=-1
      settings: Save2DSignal=2-D array (concatenate along first dimension)
  Total Torque : MATLAB Function  TreatAsAtomicUnit=on
  Torq : Outport
  wires:
  r/1 -> Product1/2, Total Torque/1(r)
  Product1/1 -> To Workspace7/1, Total Torque/2(dQ)
  dD/1 -> Sum1/2
  Total Torque/1(Torq) -> To Workspace1/1, Torq/1
  Sum1/1 -> Product1/1
  dL/1 -> Sum1/1

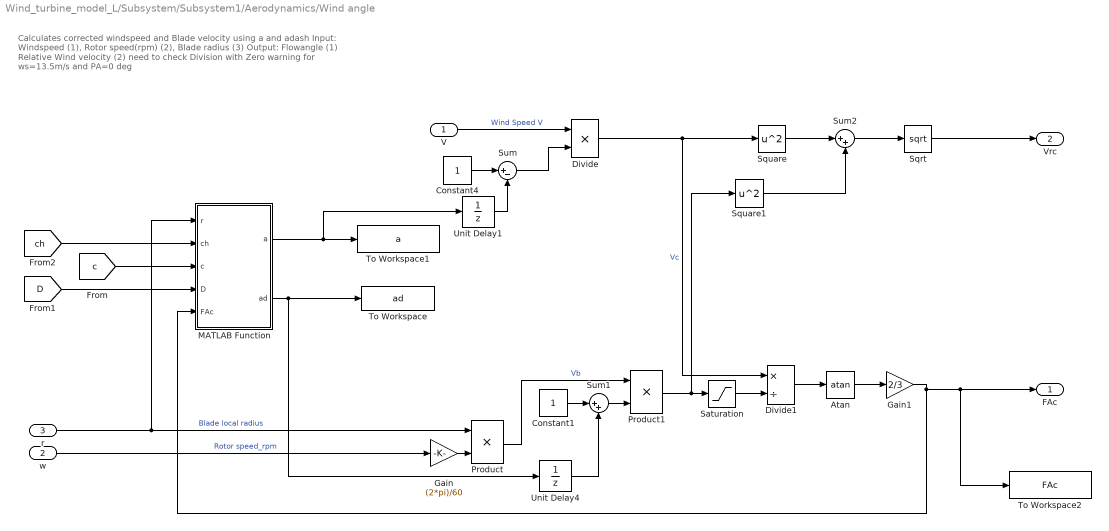
== system Wind_turbine_model_L/Subsystem/Subsystem1/Aerodynamics/Wind angle ==
  note: Calculates corrected windspeed and Blade velocity using a and adash
      |
      | Input:
      | Windspeed (1),
      | Rotor speed(rpm) (2),
      | Blade radius (3)
      |
      | Output:
      | Flowangle (1)
      | Relative Wind velocity (2)
      |
      | need to check Division with Zero warning for ws=13.5m/s and PA=0 deg
  V : Inport
  w : Inport  Port=2
  r : Inport  Port=3
  Atan : Trigonometry  Operator=atan
  Constant1 : Constant
  Constant4 : Constant
  Divide : Product  Inputs=**
  Divide1 : Product  Inputs=*/
  Gain : Gain  Gain=(2*pi)/60
  Gain1 : Gain  Gain=2/3
  MATLAB Function : MATLAB Function  TreatAsAtomicUnit=on
  Product : Product
  Product1 : Product
  Saturation : Saturate  UpperLimit=1000  LowerLimit=0.5
  Sqrt : Sqrt  SaturateOnIntegerOverflow=on
  Square : Math  Operator=square  SaturateOnIntegerOverflow=on
  Square1 : Math  Operator=square  SaturateOnIntegerOverflow=on
  Sum : Sum  Inputs=|+-
  Sum1 : Sum  Inputs=|++
  Sum2 : Sum  Inputs=|++
  To Workspace : ToWorkspace  VariableName=ad  SampleTime=-1
      settings: Save2DSignal=2-D array (concatenate along first dimension)
  To Workspace1 : ToWorkspace  VariableName=a  SampleTime=-1
      settings: Save2DSignal=2-D array (concatenate along first dimension)
  To Workspace2 : ToWorkspace  VariableName=FAc  SampleTime=-1
      settings: Save2DSignal=2-D array (concatenate along first dimension)
  Unit Delay1 : UnitDelay  SampleTime=-1  HasFrameUpgradeWarning=on
  Unit Delay4 : UnitDelay  SampleTime=-1  HasFrameUpgradeWarning=on
  FAc : Outport
  Vrc : Outport  Port=2
  wires:
  Gain/1 -> Product/2
  Sum/1 -> Divide/2
  Constant4/1 -> Sum/1
  Divide1/1 -> Atan/1
  w/1 -> Gain/1  "Rotor speed_rpm"
  Constant1/1 -> Sum1/1
  Sum1/1 -> Product1/2
  r/1 -> Product/1, MATLAB Function/1(r)  "Blade local radius"
  Square/1 -> Sum2/1
  Square1/1 -> Sum2/2
  Sum2/1 -> Sqrt/1
  Sqrt/1 -> Vrc/1
  [ch] -> MATLAB Function/2(ch)
  MATLAB Function/2(ad) -> Unit Delay4/1, To Workspace/1
  MATLAB Function/1(a) -> Unit Delay1/1, To Workspace1/1
  V/1 -> Divide/1  "Wind Speed V"
  Divide/1 -> Square/1, Divide1/1  "Vc"
  Product/1 -> Product1/1  "Vb"
  Product1/1 -> Saturation/1, Square1/1
  Atan/1 -> Gain1/1
  Gain1/1 -> To Workspace2/1, FAc/1, MATLAB Function/5(FAc)
  Unit Delay1/1 -> Sum/2
  Unit Delay4/1 -> Sum1/2
  [D] -> MATLAB Function/4(D)
  [c] -> MATLAB Function/3(c)
  Saturation/1 -> Divide1/2

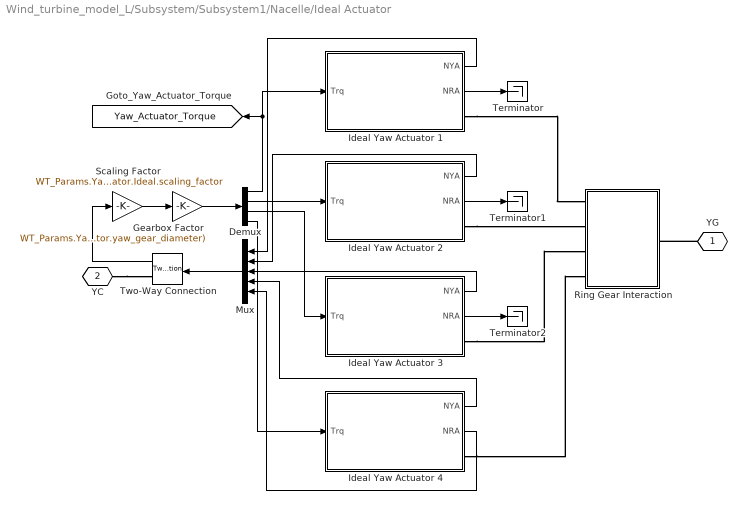
== system Wind_turbine_model_L/Subsystem/Subsystem1/Nacelle/Ideal Actuator ==
  Demux : Demux
  Gearbox Factor : Gain  Gain=WT_Params.Yaw_Actuator.p_gear_rato_step_1*WT_Params.Yaw_Actuator.p_gear_rato_step_2*WT_Params.Yaw_Actuator.p_gear_rato_step_3*WT_Params.Yaw_Actuator.p_gear_rato_step_4*(WT_Params.Yaw_Actuator.yaw_ring_diameter/WT_Params.Yaw_Actuator.yaw_gear_diameter)
  Ideal Yaw Actuator 1 : Subsystem  AncestorBlock=Yaw_Ideal_Actuator_Lib/Ideal Yaw Actuator 1
      mask Display: image('Yaw_Ideal_Actuator_Horizontal_IMAGE.jpg');
  Ideal Yaw Actuator 2 : Subsystem  AncestorBlock=Yaw_Ideal_Actuator_Lib/Ideal Yaw Actuator 1
      mask Display: image('Yaw_Ideal_Actuator_Horizontal_IMAGE.jpg');
  Ideal Yaw Actuator 3 : Subsystem  AncestorBlock=Yaw_Ideal_Actuator_Lib/Ideal Yaw Actuator 1
      mask Display: image('Yaw_Ideal_Actuator_Horizontal_IMAGE.jpg');
  Ideal Yaw Actuator 4 : Subsystem  AncestorBlock=Yaw_Ideal_Actuator_Lib/Ideal Yaw Actuator 1
      mask Display: image('Yaw_Ideal_Actuator_Horizontal_IMAGE.jpg');
  Mux : Mux  Inputs=5
  Ring Gear Interaction : Subsystem
  Scaling Factor : Gain  Gain=WT_Params.Yaw_Actuator.Ideal.scaling_factor
  Terminator : Terminator
  Terminator1 : Terminator
  Terminator2 : Terminator
  Two-Way Connection : TwoWayConnection
  YG : PMIOPort  Tag=PMCPort  Side=Left
  YC : PMIOPort  Tag=PMCPort  Port=2  Side=Right
  tag scope: Yaw_Actuator_Torque=global
  wires:
  Mux/1 -> Two-Way Connection/1
  Gearbox Factor/1 -> Demux/1
  Ideal Yaw Actuator 1/1(NYA) -> Mux/1
  Two-Way Connection/1 -> Scaling Factor/1
  Demux/1 -> Ideal Yaw Actuator 1/1(Trq), [Yaw_Actuator_Torque]
  Ideal Yaw Actuator 1/2(NRA) -> Terminator/1
  Ideal Yaw Actuator 2/2(NRA) -> Terminator1/1
  Ideal Yaw Actuator 3/2(NRA) -> Terminator2/1
  Ideal Yaw Actuator 4/2(NRA) -> Mux/5
  Demux/2 -> Ideal Yaw Actuator 2/1(Trq)
  Demux/3 -> Ideal Yaw Actuator 3/1(Trq)
  Demux/4 -> Ideal Yaw Actuator 4/1(Trq)
  Ideal Yaw Actuator 2/1(NYA) -> Mux/2
  Ideal Yaw Actuator 3/1(NYA) -> Mux/3
  Ideal Yaw Actuator 4/1(NYA) -> Mux/4
  Scaling Factor/1 -> Gearbox Factor/1
  connections:
  YC/RConn1 -- Two-Way Connection/RConn1
  YG/RConn1 -- Ring Gear Interaction/RConn1
  Ideal Yaw Actuator 1/RConn1 -- Ring Gear Interaction/LConn1
  Ideal Yaw Actuator 2/RConn1 -- Ring Gear Interaction/LConn2
  Ideal Yaw Actuator 3/RConn1 -- Ring Gear Interaction/LConn3
  Ideal Yaw Actuator 4/RConn1 -- Ring Gear Interaction/LConn4

== system Wind_turbine_model_L/Subsystem/Yaw Controller/Yaw Controller/PI Controller Nacelle Yaw ==
  e : Inport
  Integral Gain : Gain  Gain=WT_Params.Yaw_Controller.I_Gain  SaturateOnIntegerOverflow=on  OutDataTypeStr=Inherit: Same as input  ParamDataTypeStr=Inherit: Same as input
  Integrator : Integrator  LimitOutput=on  UpperSaturationLimit=WT_Params.Yaw_Actuator.max_yaw_rate  LowerSaturationLimit=-WT_Params.Yaw_Actuator.max_yaw_rate
  Proportional Gain : Gain  Gain=WT_Params.Yaw_Controller.P_Gain  SaturateOnIntegerOverflow=on  OutDataTypeStr=Inherit: Same as input  ParamDataTypeStr=Inherit: Same as input
  Sum : Sum  Inputs=++|  InputSameDT=on  SaturateOnIntegerOverflow=on  OutDataTypeStr=Inherit: Same as first input
  u : Outport  InitialOutput=0  VectorParamsAs1DForOutWhenUnconnected=off
  wires:
  Integral Gain/1 -> Integrator/1
  Proportional Gain/1 -> Sum/1
  Integrator/1 -> Sum/2
  e/1 -> Proportional Gain/1, Integral Gain/1
  Sum/1 -> u/1

== system Wind_turbine_model_L/Subsystem/Yaw Controller/Yaw Controller/PI Controller Nacelle Yaw Rate ==
  e : Inport
  Integral Gain : Gain  Gain=WT_Params.Yaw_Controller.Yaw_Rate.I_Gain  SaturateOnIntegerOverflow=on  OutDataTypeStr=Inherit: Same as input  ParamDataTypeStr=Inherit: Same as input
  Integrator : Integrator  LimitOutput=on  UpperSaturationLimit=max(WT_Params.Yaw_Actuator.Motor.max_torque_vector)  LowerSaturationLimit=-max(WT_Params.Yaw_Actuator.Motor.max_torque_vector)
  Proportional Gain : Gain  Gain=WT_Params.Yaw_Controller.Yaw_Rate.P_Gain  SaturateOnIntegerOverflow=on  OutDataTypeStr=Inherit: Same as input  ParamDataTypeStr=Inherit: Same as input
  Sum : Sum  Inputs=++|  InputSameDT=on  SaturateOnIntegerOverflow=on  OutDataTypeStr=Inherit: Same as first input
  u : Outport  InitialOutput=0  VectorParamsAs1DForOutWhenUnconnected=off
  wires:
  Sum/1 -> u/1
  e/1 -> Integral Gain/1, Proportional Gain/1
  Integrator/1 -> Sum/2
  Proportional Gain/1 -> Sum/1
  Integral Gain/1 -> Integrator/1

== system Wind_turbine_model_L/Subsystem/Subsystem1/Aerodynamics/LookUp_Table/FFAW3_241(9to17) ==
  AOA : Inport
  Cd : ToWorkspace  Commented=on  VariableName=Cd3  SampleTime=-1
      settings: Save2DSignal=2-D array (concatenate along first dimension)
  Cl : ToWorkspace  Commented=on  VariableName=Cl3  SampleTime=-1
      settings: Save2DSignal=2-D array (concatenate along first dimension)
  Drag Polar : Lookup_n-D  NumberOfTableDimensions=1  BreakpointsForDimension1=|  Table=|  InternalRulePriority=Speed  RndMeth=Simplest  InputSameDT=on
      BreakpointsForDimension1=|
      | [-4.66442953
      | -3.951342282
      | -3.36409396
      | -2.609060403
      | -1.895973154
      | -1.266778523
      | -0.511744966
      | 0.033557047
      | 0.830536913
      | 1.543624161
      | 2.088926174
      | 2.718120805
      | 3.55704698
      | 4.270134228
      | 5.067114094
      | 6.031879195
      | 6.954697987
      | 7.583892617
      | 8.296979866
      | 8.968120805
      | 9.639261745
      | 10.26845638
      | 11.23322148
      | 11.90436242
      | 12.44966443
      | 12.95302013
      | 13.70805369
      | 14.2533557
      | 14.75671141
      | 15.26006711
      | 15.76342282
      | 16.01510067]
      Table=|
      | [0.010843373
      | 0.010240964
      | 0.009939759
      | 0.010240964
      | 0.009638554
      | 0.009939759
      | 0.009337349
      | 0.009939759
      | 0.009939759
      | 0.010542169
      | 0.010542169
      | 0.011144578
      | 0.011144578
      | 0.011746988
      | 0.012349398
      | 0.012650602
      | 0.014156627
      | 0.014457831
      | 0.014759036
      | 0.016566265
      | 0.017168675
      | 0.017771084
      | 0.020180723
      | 0.021385542
      | 0.022289157
      | 0.023192771
      | 0.026204819
      | 0.028012048
      | 0.031024096
      | 0.034337349
      | 0.039457831
      | 0.041566265]
  Lift Polar : Lookup_n-D  NumberOfTableDimensions=1  BreakpointsForDimension1=|  Table=|  InternalRulePriority=Speed  RndMeth=Simplest  InputSameDT=on
      BreakpointsForDimension1=|
      | [0.165837479
      | 0.870646766
      | 1.451077944
      | 2.031509121
      | 2.529021559
      | 3.109452736
      | 3.565505804
      | 4.104477612
      | 4.60199005
      | 5.016583748
      | 5.679933665
      | 6.343283582
      | 6.92371476
      | 7.587064677
      | 8.084577114
      | 8.830845771
      | 9.577114428
      | 9.950248756
      | 10.61359867
      | 11.35986733
      | 12.10613599
      | 12.89386401
      | 13.64013267
      | 14.51077944
      | 15.46434494
      | 16.12769486
      | 16.83250415
      | 17.66169154
      | 18.44941957
      | 19.32006633
      | 20.02487562
      | 20.77114428
      | 21.51741294
      | 22.30514096
      | 22.96849088
      | 23.79767828
      | 24.25373134
      | 24.66832504]
      Table=|
      | [0.238095238
      | 0.285714286
      | 0.357142857
      | 0.416666667
      | 0.5
      | 0.55952381
      | 0.607142857
      | 0.654761905
      | 0.720238095
      | 0.785714286
      | 0.845238095
      | 0.922619048
      | 1
      | 1.035714286
      | 1.107142857
      | 1.166666667
      | 1.244047619
      | 1.297619048
      | 1.357142857
      | 1.398809524
      | 1.44047619
      | 1.517857143
      | 1.523809524
      | 1.458333333
      | 1.43452381
      | 1.422619048
      | 1.416666667
      | 1.410714286
      | 1.392857143
      | 1.380952381
      | 1.357142857
      | 1.345238095
      | 1.30952381
      | 1.297619048
      | 1.279761905
      | 1.279761905
      | 1.261904762
      | 1.214285714]
  Output : Outport
  Output1 : Outport  Port=2
  wires:
  AOA/1 -> Drag Polar/1, Lift Polar/1
  Drag Polar/1 -> Output1/1
  Lift Polar/1 -> Output/1
